simulink model "L0506"  (Simulink 10.2)
settings: Solver=VariableStepAuto  StartTime=0.0  StopTime=15  RelTol=1e-3
values from neighbouring files (symbols this model uses):
  xInitial = [1 1]    [Lab0506.m]
settings Model: Creator=Ranci  LastModifiedBy=Ranci
settings DataIOCC: LoadExternalInput=on  LoadInitialState=on  SaveFormat=StructureWithTime  SignalLoggingSaveFormat=Dataset  ReturnWorkspaceOutputs=on
settings OptimizationCC: LifeSpan=auto
settings DebuggingCC: UnderspecifiedInitializationDetection=Simplified  MergeDetectMultiDrivingBlocksExec=error  FcnCallInpInsideContextMsg=error  SFUnexpectedBacktrackingDiag=error  SFNoUnconditionalDefaultTransitionDiag=error  SFExecutionAtInitializationDiag=warning  ArithmeticOperatorsInVariantConditions=error
settings HardwareCC: ProdBitPerPointer=64  ProdBitPerSizeT=64  ProdBitPerPtrDiffT=64  ProdLargestAtomicFloat=Float  ProdIntDivRoundTo=Zero  ProdEndianess=LittleEndian  ProdWordSize=64  ProdHWDeviceType=Intel->x86-64 (Windows64)
settings ModelReferenceCC: PropagateSignalLabelsOutOfModel=on
settings SFSimCC: SimUseLocalCustomCode=on  CustomCodeUndefinedFunction=FilterOut
settings RTWCC: RTWUseLocalCustomCode=on
settings CodeAppCC: StateflowObjectComments=off
settings GRTTargetCC: TargetLangStandard=C99 (ISO)  CombineOutputUpdateFcns=on  GRTInterface=off
settings ConfigComp: CovMetricSettings=dwe  CovSaveCumulativeToWorkspaceVar=off  CovSaveSingleToWorkspaceVar=off  CovExternalEMLEnable=on

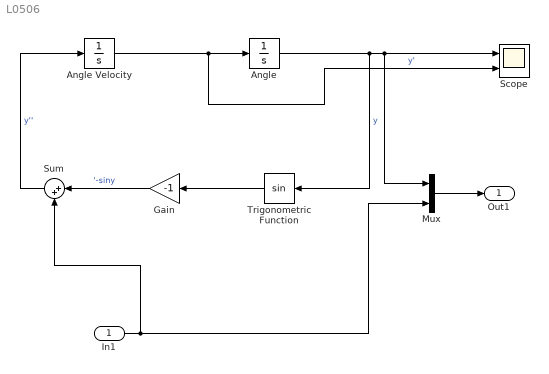
== system L0506 ==
  In1 : Inport  PortDimensions=1
  Angle : Integrator  InitialCondition=xInitial(2)
  Angle Velocity : Integrator  InitialCondition=xInitial(1)
  Gain : Gain  Gain=-1
  Mux : Mux  Inputs=2
  Scope : Scope  NumInputPorts=2
  Sum : Sum  Inputs=|++
  Trigonometric Function : Trigonometry
  Out1 : Outport  SignalName=Data  PortDimensions=2
  wires:
  Angle Velocity/1 -> Scope/2, Angle/1  "y'"
  Angle/1 -> Trigonometric Function/1, Scope/1, Mux/1  "y"
  Trigonometric Function/1 -> Gain/1
  In1/1 -> Mux/2, Sum/2
  Gain/1 -> Sum/1  "'-siny"
  Sum/1 -> Angle Velocity/1  "y''"
  Mux/1 -> Out1/1
